simulink model "TC1_MappingSingle"  (R2016a)
settings: Solver=FixedStepAuto  StartTime=0.0  StopTime=10.0  RelTol=1e-3
model workspace: external: MAT-File TC1_MappingSingle.mat (data not in the file)
values from neighbouring files (symbols this model uses):
  dripTestCasedripX = 0.19576554744588748    (= 0.195765547446)    [TC1_MappingSingle_params.m]
  dripTestCasedripY = 1.0533299169351737    (= 1.05332991694)    [TC1_MappingSingle_params.m]
settings Model: Creator=Josef  LastModifiedBy=Josef
settings GRTTargetCC: GeneratePreprocessorConditionals=Use local settings

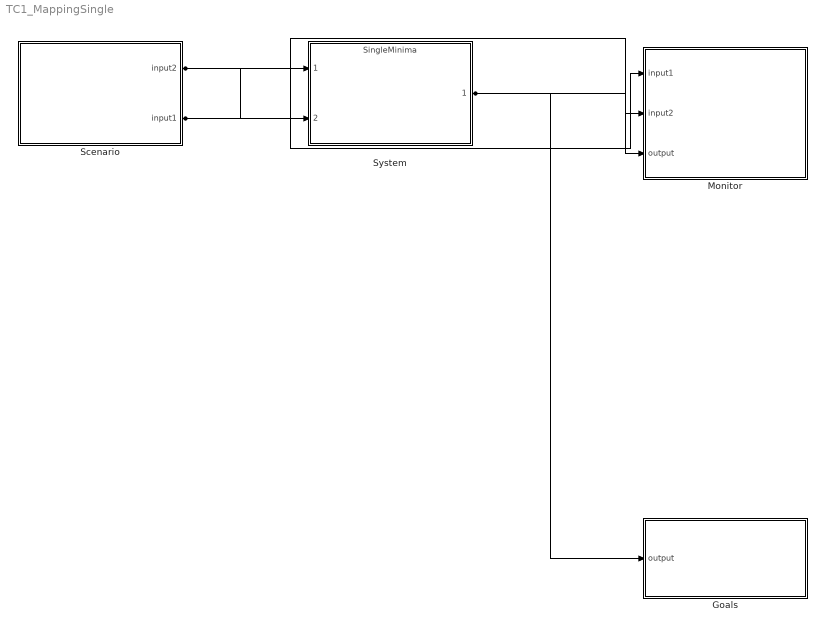
== system TC1_MappingSingle ==
  Goals : Subsystem
  Monitor : Subsystem
  Scenario : Subsystem
  System : ModelReference  ModelNameDialog=SingleMinima  SimulationMode=Normal  ModelReferenceVersion=1.12
  wires:
  Scenario/2(input1) -> System/1, Monitor/1(input1)
  Scenario/1(input2) -> System/2, Monitor/2(input2)
  System/1 -> Monitor/3(output), Goals/1(output)

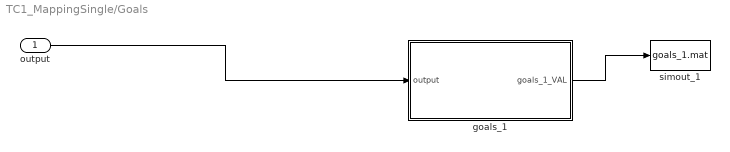
== system TC1_MappingSingle/Goals ==
  output : Inport
  goals_1 : Subsystem
  simout_1 : ToFile  Filename=goals_1.mat  MatrixName=goals_1  SaveFormat=Timeseries
  wires:
  output/1 -> goals_1/1(output)
  goals_1/1(goals_1_VAL) -> simout_1/1

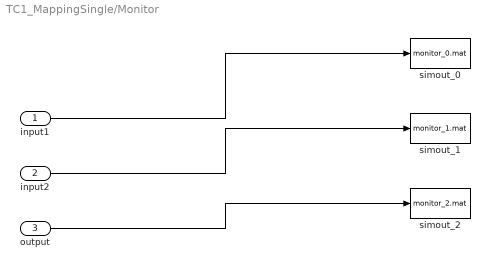
== system TC1_MappingSingle/Monitor ==
  input1 : Inport
  input2 : Inport  Port=2
  output : Inport  Port=3
  simout_0 : ToFile  Filename=monitor_0.mat  MatrixName=input1  SaveFormat=Timeseries
  simout_1 : ToFile  Filename=monitor_1.mat  MatrixName=input2  SaveFormat=Timeseries
  simout_2 : ToFile  Filename=monitor_2.mat  MatrixName=output  SaveFormat=Timeseries
  wires:
  input1/1 -> simout_0/1
  input2/1 -> simout_1/1
  output/1 -> simout_2/1

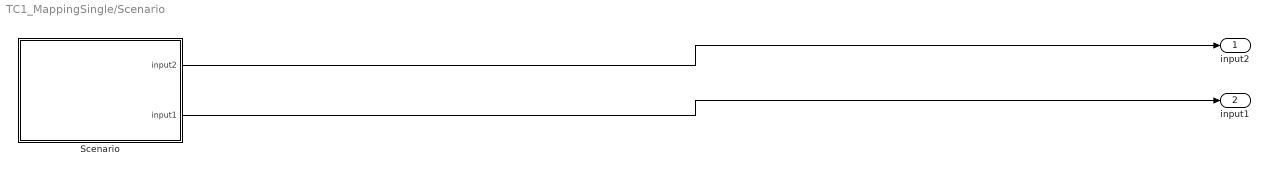
== system TC1_MappingSingle/Scenario ==
  Scenario : Stateflow chart  TreatAsAtomicUnit=on
  input2 : Outport
  input1 : Outport  Port=2
  wires:
  Scenario/2(input1) -> input1/1
  Scenario/1(input2) -> input2/1

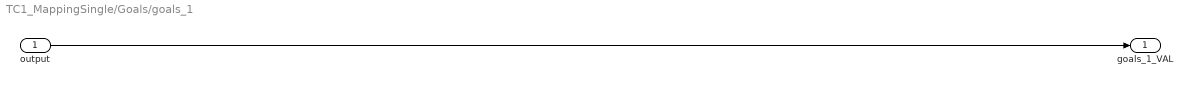
== system TC1_MappingSingle/Goals/goals_1 ==
  output : Inport
  goals_1_VAL : Outport
  wires:
  output/1 -> goals_1_VAL/1

== stateflow chart TC1_MappingSingle/Scenario/Scenario ==
  state Act_A_Step1
    entry: input1 = dripTestCasedripX;
    entry: input2 = dripTestCasedripY;
  (default) -> Act_A_Step1
  data: input2 output; input1 output; dripTestCasedripY parameter; dripTestCasedripX parameter
